simulink model "LongitudinalControl"  (R2018b)
settings: Solver=FixedStepAuto  StartTime=0.0  StopTime=100  FixedStep=0.001  RelTol=5e-3
model workspace (MAT data in the model file):
  A_mu = 10
  AxlIxx = 62.3745166667
  AxlM = 160
  B_reff = 8.386
  Cps = 2
  Cps1 = 2
  Cz = 7766.25
  Cz1 = 5565.2246438
  CzWhlAxl = 11490.971257
  DCT_Param : struct (value not decoded)
  DCT_Param1 : struct (value not decoded)
  D_reff = 0.25826
  Downshift_Speeds = [9.5625 12.9375 16.3125 19.6875 23.0625 26.4375 29.8125 33.1875 36.5625 39.9375 43.3125 46.6875 ... (28 elements, 4x7)]
  Downshift_Speeds1 = [9.5625 12.9375 16.3125 19.6875 23.0625 26.4375 29.8125 33.1875 36.5625 39.9375 43.3125 46.6875 ... (28 elements, 4x7)]
  F0z = [6086.4 4324.8]
  F0z1 = [2886 2907]
  F0zWhlAxl = 2907
  F_reff = 0.07394
  F_zmax = 10000
  F_zmin = 100
  F_zo = 4000
  Hmax = 0.25
  Kz = 48000
  Kz1 = 52451.0065793
  KzWhlAxl = 138031.612078
  MF : struct (value not decoded)
  NCyl = 6
  NCyl1 = 6
  NE_VEC = [800 1200 1600 2000 2400 2800 3200 3600 4000 4400 4800]
  Pedal_Positions = [0.1 0.4 0.5 0.9]
  Pedal_Positions1 = [0.1 0.4 0.5 0.9]
  Pstd = 101325
  Pstd1 = 101325
  Rair = 287
  Rair1 = 287
  SUS : struct (value not decoded)
  SUS1 : struct (value not decoded)
  MCOS : class17 (value not decoded)
  MCOS : class17 (value not decoded)
  MCOS : class17 (value not decoded)
  Trans : struct (value not decoded)
  Trans1 : struct (value not decoded)
  Tstd = 293.15
  Tstd1 = 293.15
  Upshift_Speeds = [12.9375 16.3125 19.6875 33 26.4375 29.8125 33.1875 52.5 39.9375 43.3125 46.6875 77.25 ... (28 elements, 4x7)]
  Upshift_Speeds1 = [12.9375 16.3125 19.6875 33 26.4375 29.8125 33.1875 52.5 39.9375 43.3125 46.6875 77.25 ... (28 elements, 4x7)]
  VEH : struct (value not decoded)
  VEH1 : struct (value not decoded)
  V_o = 16.7
  V_xlow = 1
  Vd = 0.00346
  Vd1 = 0.00346
  WH : struct (value not decoded)
  WH1 : struct (value not decoded)
  a = 1.4
  alpha_max = 1.5
  alpha_min = -1.5
  b = 1.8
  c_zo = 209651
  dt3D = 0.05
  epsilon = 0.1
  f_air = [0 0 0 0 0 0 0 0 0 0 0 0 ... (256 elements, 16x16)]
  f_air1 = [0 0 0 0 0 0 0 0 0 0 0 0 ... (256 elements, 16x16)]
  f_co = [0 0 0 0 0 0 0 0 0 0 0 0 ... (256 elements, 16x16)]
  f_co1 = [0 0 0 0 0 0 0 0 0 0 0 0 ... (256 elements, 16x16)]
  f_co2 = [0 0 0 0 0 0 0 0 0 0 0 0 ... (256 elements, 16x16)]
  f_co3 = [0 0 0 0 0 0 0 0 0 0 0 0 ... (256 elements, 16x16)]
  f_eff = [352.135682859 352.135682859 320.724378192 303.655312657 295.930136708 291.240087194 291.240271258 291.240312459 291.240275452 291.240198499 291.240100781 291.240018769 ... (256 elements, 16x16)]
  f_eff1 = [352.135682859 352.135682859 320.724378192 303.655312657 295.930136708 291.240087194 291.240271258 291.240312459 291.240275452 291.240198499 291.240100781 291.240018769 ... (256 elements, 16x16)]
  f_fuel = [0 0 0 0 0 0 0 0 0 0 0 0 ... (256 elements, 16x16)]
  f_fuel1 = [0 0 0 0 0 0 0 0 0 0 0 0 ... (256 elements, 16x16)]
  f_hc = [0 0 0 0 0 0 0 0 0 0 0 0 ... (256 elements, 16x16)]
  f_hc1 = [0 0 0 0 0 0 0 0 0 0 0 0 ... (256 elements, 16x16)]
  f_nox = [0 0 0 0 0 0 0 0 0 0 0 0 ... (256 elements, 16x16)]
  f_nox1 = [0 0 0 0 0 0 0 0 0 0 0 0 ... (256 elements, 16x16)]
  f_pm = [0 0 0 0 0 0 0 0 0 0 0 0 ... (256 elements, 16x16)]
  f_pm1 = [0 0 0 0 0 0 0 0 0 0 0 0 ... (256 elements, 16x16)]
  f_susp_axl_bp = [1 2]
  f_susp_axl_bp1 = [1 2]
  f_susp_dz_bp = [-4 -0.14 -0.13 -0.12 -0.11 -0.1 -0.09 -0.08 -0.07 -0.06 -0.05 -0.04 ... (31 elements, 1x31)]
  f_susp_dz_bp1 = [-0.325022776267 -0.315022776267 -0.305022776267 -0.205022776267 -0.105022776267 -0.00502277626717 0.0949772237328 0.194977223733 0.204977223733 0.214977223733]
  f_susp_dzdot_bp = [-4 -0.14 -0.13 -0.12 -0.11 -0.1 -0.09 -0.08 -0.07 -0.06 -0.05 -0.04 ... (31 elements, 1x31)]
  f_susp_dzdot_bp1 = [-3 -0.3 -0.2 -0.1 0 0.1 0.2 0.3 3]
  f_susp_fmz = [-213379.591456 -28099.591456 -27619.591456 -27139.591456 -26659.591456 -26179.591456 -25699.591456 -25219.591456 -24739.591456 -24259.591456 -23779.591456 -23299.591456 ... (468968 elements, 31x31x61x2x4)]
  f_susp_fmz1 = [-144070.391448 -93629.24037 -75929.1118915 -20630.5828179 -15385.48216 -10140.3815021 -4895.28084414 349.819813785 -31916.3973792 18437.6709544 -83996.1993354 -33555.0482577 ... (43920 elements, 10x9x61x2x4)]
  f_susp_geom = [-0.832564012244 0.043269987756 0.045538987756 0.047807987756 0.050076987756 0.052345987756 0.054614987756 0.056883987756 0.059152987756 0.061421987756 0.063690987756 0.065959987756 ... (11346 elements, 31x61x2x3)]
  f_susp_geom1 = [0 0 0 0 0 0 0 0 0 0 0 0 ... (3660 elements, 10x61x2x3)]
  f_susp_strgdelta_bp = [-0.523598775598 -0.506145483078 -0.488692190558 -0.471238898038 -0.453785605519 -0.436332312999 -0.418879020479 -0.401425727959 -0.383972435439 -0.366519142919 -0.349065850399 -0.331612557879 ... (61 elements, 1x61)]
  f_susp_strgdelta_bp1 = [-0.523598775598 -0.506145483078 -0.488692190558 -0.471238898038 -0.453785605519 -0.436332312999 -0.418879020479 -0.401425727959 -0.383972435439 -0.366519142919 -0.349065850399 -0.331612557879 ... (61 elements, 1x61)]
  f_tbrake = [0 76.8593923996 105.140482948 131.533638111 157.926793274 176.658631717 176.65727296 176.656856686 176.656879077 176.657093756 176.657404516 176.65772406 ... (256 elements, 16x16)]
  f_tbrake1 = [0 76.8593923996 105.140482948 131.533638111 157.926793274 176.658631717 176.65727296 176.656856686 176.656879077 176.657093756 176.657404516 176.65772406 ... (256 elements, 16x16)]
  f_tbrake_n_bpt = [0 649.519052838 912.419621844 1175.32019085 1438.22075986 1701.12132886 1964.02189787 2226.92246687 2489.82303588 2752.72360489 3015.62417389 3278.5247429 ... (16 elements, 1x16)]
  f_tbrake_n_bpt1 = [0 649.519052838 912.419621844 1175.32019085 1438.22075986 1701.12132886 1964.02189787 2226.92246687 2489.82303588 2752.72360489 3015.62417389 3278.5247429 ... (16 elements, 1x16)]
  f_tbrake_t_bpt = [0 34.6410161514 61.0341713143 87.4273264773 113.82048164 140.213636803 166.606791966 192.999947129 219.393102292 245.786257455 272.179412618 298.572567781 ... (16 elements, 1x16)]
  f_tbrake_t_bpt1 = [0 34.6410161514 61.0341713143 87.4273264773 113.82048164 140.213636803 166.606791966 192.999947129 219.393102292 245.786257455 272.179412618 298.572567781 ... (16 elements, 1x16)]
  f_texh = [766.752464599 766.752464599 786.17542386 801.679939032 884.591982581 910.574397722 910.571871054 910.570774534 910.570601632 910.570821151 910.571247242 910.571639815 ... (256 elements, 16x16)]
  f_texh1 = [766.752464599 766.752464599 786.17542386 801.679939032 884.591982581 910.574397722 910.571871054 910.570774534 910.570601632 910.570821151 910.571247242 910.571639815 ... (256 elements, 16x16)]
  f_twc_eff_co = [0.17 0.25 0.45 0.99 0.99 0.99 0.99]
  f_twc_eff_co1 = [0.17 0.25 0.45 0.99 0.99 0.99 0.99]
  f_twc_eff_hc = [0.21 0.375 0.75 0.98 0.98 0.98 0.98]
  f_twc_eff_hc1 = [0.21 0.375 0.75 0.98 0.98 0.98 0.98]
  f_twc_eff_lam = [0.909090909 0.944055944 0.979020979 1 1.013986014 1.048951049 1.083916084]
  f_twc_eff_lam1 = [0.909090909 0.944055944 0.979020979 1 1.013986014 1.048951049 1.083916084]
  f_twc_eff_nox = [0.98 0.98 0.98 0.97 0.05 0.02 0]
  f_twc_eff_nox1 = [0.98 0.98 0.98 0.97 0.05 0.02 0]
  h = 0.134
  h1 = 0.5
  h2 = 0.134
  k_z = 50
  kappa_max = 1.5
  kappa_min = -1.5
  lam_Cx = 1
  lam_Cy = 1
  lam_Cz = 1
  lam_Ex = 1
  lam_Ey = 1
  lam_F_zo = 1
  lam_Hx = 1
  lam_Hy = 1
  lam_Kxkappa = 1
  lam_Kyalpha = 1
  lam_Kygamma = 1
  lam_Kzgamma = 1
  lam_Mr = 1
  lam_Mx = 1
  lam_My = 1
  lam_S = 1
  lam_VMx = 1
  lam_Vx = 1
  lam_Vy = 1
  lam_Vykappa = 1
  lam_muV = 0
  lam_mux = 1
  lam_muy = 1
  lam_t = 1
  lam_xalpha = 1
  lam_ykappa = 1
  numWheel = 4
  numWheel1 = 4
  p_Cx1 = 1.579
  p_Cy1 = 1.3332
  p_Dx1 = 1.0422
  p_Dx2 = -0.08285
  p_Dx3 = 0
  p_Dy1 = 0.8784
  p_Dy2 = -0.06445
  p_Dy3 = 0
  p_Ex1 = 0.11185
  p_Ex2 = 0.3127
  p_Ex3 = 0
  p_Ex4 = 0.001603
  p_Ey1 = -0.8227
  p_Ey2 = -0.6062
  p_Ey3 = 0.09825
  p_Ey4 = -6.546
  p_Ey5 = 0
  p_Fz1 = 0.7098
  p_Hx1 = 0.00021585
  p_Hx2 = 0.0011538
  p_Hy1 = -0.0018043
  p_Hy2 = 0.003518
  p_Kx1 = 21.69
  p_Kx2 = 13.774
  p_Kx3 = -0.4119
  p_Ky1 = -15.314
  p_Ky2 = 1.7044
  p_Ky3 = 0.36986
  p_Ky4 = 1.9896
  p_Ky5 = 0
  p_Ky6 = -0.9004
  p_Ky7 = -0.2328
  p_Vx1 = 1.5973e-05
  p_Vx2 = 0.0001043
  p_Vy1 = -0.006642
  p_Vy2 = 0.03597
  p_Vy3 = -0.1621
  p_Vy4 = -0.4908
  p_pmx1 = 0
  p_px1 = -0.3489
  p_px2 = 0.382
  p_px3 = -0.09634
  p_px4 = 0.06447
  p_py1 = -0.6249
  p_py2 = -0.06535
  p_py3 = -0.1668
  p_py4 = 0.2834
  p_py5 = 0
  path : struct (value not decoded)
  pio = 220000
  q_Fcx = 0
  q_Fz2 = 15.4
  q_Fzy = 0
  q_reo = 0.9974
  q_sx1 = -0.007764
  q_sx10 = 0.2824
  q_sx11 = 5.349
  q_sx12 = 0
  q_sx13 = 0
  q_sx14 = 0
  q_sx2 = 1.1915
  q_sx3 = 0.013948
  q_sx4 = 4.912
  q_sx5 = 1.02
  q_sx6 = 22.83
  q_sx7 = 0.7104
  q_sx8 = -0.023393
  q_sx9 = 0.6581
  q_sy1 = 0.00702
  q_sy2 = 0
  q_sy3 = 0.001515
  q_sy4 = 8.514e-05
  q_sy5 = 0
  q_sy6 = 0
  q_sy7 = 0.9008
  q_sy8 = -0.4089
  q_v1 = 0.0007742
  q_v2 = 0.04667
  r_Bx1 = 12.531
  r_Bx2 = 9.532
  r_Bx3 = 0
  r_By1 = 10.615
  r_By2 = 7.705
  r_By3 = 3.433e-06
  r_By4 = 0
  r_Cx1 = 1.019
  r_Cy1 = 1.0585
  r_Ex1 = -0.4487
  r_Ex2 = -0.4726
  r_Ey1 = 0.3132
  r_Ey2 = 7.63e-06
  r_Hx1 = 0.0002374
  r_Hy1 = 0.011646
  r_Hy2 = 7.63e-06
  r_Vy1 = 0.05654
  r_Vy2 = 7.63e-06
  r_Vy3 = 0
  r_Vy4 = 99.9
  r_Vy5 = 2
  r_Vy6 = 15.814
  r_o = 0.3135
  vehWidth = 2
  w = 1
symbols that are objects in the model workspace (value not decoded): Trans, VEH
undefined symbols (not defined in the file): Angular, Linear, sigbuilder_block
libraries: robotlib x31, autolibutils x10, autolibshared x8, vehdynlibsuspension x7, simulink x5, vehdynlibtire x4, autolibsharedcoupling x3, vehdynlibtirecommon x3, sharedtransform x3, sim3dlib x1, vehdynlibsteering x1, autolibshareddiff x1
(part 2 of 11)

== system LongitudinalControl/Controllers ==
  note: Converts to Acceleration to Torque
      | (probably in N-m, needs to check)
  note: Determines Gear Switching
  note: Calculates Brake Pressure
      | (probably in Pascal, needs to check)
  Driver : Inport
  VehFdbk : Inport  Port=2
  Active Differential Control : Subsystem  VariantControlMode=Label  Variant=on  LabelModeActiveChoice=0
  Blank Message1 : robotlib/Blank Message  messageClass=Message  entityType=geometry_msgs/Wrench  messageType=geometry_msgs/Wrench  SampleTime=inf
      settings: SourceProductBaseCode=RO
  Blank Message2 : robotlib/Blank Message  messageClass=Message  entityType=std_msgs/Int8  messageType=std_msgs/Int8  SampleTime=inf
      settings: SourceProductBaseCode=RO
  Brake Controller : Subsystem
  Bus Assignment1 : BusAssignment  AssignedSignals=Torque.Z
  Bus Assignment2 : BusAssignment  AssignedSignals=Data
  Bus Creator{,1..2,4} (4 alike) : BusCreator  Inputs=1
  Bus Creator3 : BusCreator  Inputs=4
  Bus Selector : BusSelector  OutputSignals=Body.xdot,Wheels.kappa,Body.r
  Bus Selector1 : BusSelector  OutputSignals=Driveline.EngSpd,Driveline.PropShftSpd
  Bus Selector2 : BusSelector  OutputSignals=Accel,Brake
  Bus Selector3 : BusSelector  OutputSignals=Steer
  Engine Control Unit (ECU) : Subsystem
  Max : MinMax  Function=max  Inputs=2
  Publish1 : robotlib/Publish  topicSource=Specify your own  topic=engine_torque_cmd  messageType=geometry_msgs/Wrench  messageQueueLength=1
      settings: SourceProductBaseCode=RO
  Publish2 : robotlib/Publish  topicSource=Specify your own  topic=gear_cmd  messageType=std_msgs/Int8  messageQueueLength=1
      settings: SourceProductBaseCode=RO
  Transmission Controller : Subsystem
  Controller : Outport
  wires:
  Transmission Controller/1(Gear) -> Bus Assignment2/2, Bus Creator1/1  "GearCmd"
  Bus Selector/2 -> Brake Controller/3(kappa)  "<kappa>"
  Engine Control Unit (ECU)/1(Trq Cmd) -> Max/1
  VehFdbk/1 -> Bus Selector1/1, Bus Selector/1
  Bus Selector/1 -> Brake Controller/2(xdot)  "<xdot>"
  Bus Selector1/1 -> Transmission Controller/2(EngSpd)  "<EngSpd>"
  Bus Selector1/2 -> Transmission Controller/3(PropShaftSpd)  "<PropShftSpd>"
  Driver/1 -> Bus Selector3/1, Bus Selector2/1
  Bus Selector2/1 -> Transmission Controller/1(Acc), Engine Control Unit (ECU)/1(<Accel>)  "<Accel>"
  Bus Selector2/2 -> Brake Controller/1(BrkCmd)  "<Brake>"
  Bus Creator/1 -> Bus Creator3/1  "ECU"
  Bus Creator1/1 -> Bus Creator3/2  "Transmission"
  Bus Creator2/1 -> Bus Creator3/3  "Brake"
  Bus Creator3/1 -> Controller/1  "Controller"
  Bus Creator4/1 -> Bus Creator3/4  "Diff"
  Active Differential Control/1(DiffPrsCmd) -> Bus Creator4/1  "PrsCmd"
  Bus Selector3/1 -> Active Differential Control/2(Steer)  "<Steer>"
  Active Differential Control/2(TrqCmd) -> [DiffTrqCmd]
  Max/1 -> Bus Assignment1/2, Bus Creator/1  "EngTrqCmd"
  [DiffTrqCmd] -> Max/2
  Bus Selector/3 -> Active Differential Control/1(YawRate)  "<r>"
  Bus Assignment1/1 -> Publish1/1
  Blank Message1/1 -> Bus Assignment1/1
  Bus Assignment2/1 -> Publish2/1
  Blank Message2/1 -> Bus Assignment2/1
  Brake Controller/1(PCmd) -> Bus Creator2/1  "PCmd"

== system LongitudinalControl/Environment ==
  Blank Message : robotlib/Blank Message  messageClass=Message  entityType=geometry_msgs/Twist  messageType=geometry_msgs/Twist  SampleTime=inf
      settings: SourceProductBaseCode=RO
  Bus Assignment : BusAssignment  AssignedSignals=Linear.X,Linear.Y,Linear.Z
  Bus Creator1 : BusCreator  Inputs=2
  Constant3 : Constant  Value=0
  Constant4 : Constant  Value=0
  Constant5 : Constant  Value=0
  Friction : Constant  Value=ones(4,1).*1.0
  Ground Feedback : Subsystem  VariantControlMode=Label  Variant=on  LabelModeActiveChoice=0
  Publish : robotlib/Publish  topicSource=Specify your own  topic=wind  messageType=geometry_msgs/Twist  messageQueueLength=1
      settings: SourceProductBaseCode=RO
  Vector Concatenate : Concatenate  NumInputs=3
  Env : Outport
  wires:
  Constant5/1 -> Vector Concatenate/3, Bus Assignment/4  "Z"
  Vector Concatenate/1 -> Bus Creator1/1  "Wind"
  Constant3/1 -> Bus Assignment/2, Vector Concatenate/1  "X"
  Constant4/1 -> Bus Assignment/3, Vector Concatenate/2  "Y"
  Ground Feedback/1(Ground) -> Bus Creator1/2  "Gnd"
  Bus Creator1/1 -> Env/1
  Friction/1 -> Ground Feedback/1(Friction)
  Bus Assignment/1 -> Publish/1
  Blank Message/1 -> Bus Assignment/1

== system LongitudinalControl/Longitudinal Driver ==
  note: Longitudinal Driver has four inputs out of which
      | two are mandory:
      | Reference Longitudinal Velocity
      | Feedbacked velocity
      | Road Grade Angle (Optional)
      | Gear Ratio (Optional)
  VehRef : Inport
  VehFdbk : Inport  Port=2
  Blank Message : robotlib/Blank Message  messageClass=Message  entityType=geometry_msgs/Wrench  messageType=geometry_msgs/Wrench  SampleTime=inf
      settings: SourceProductBaseCode=RO
  Blank Message1 : robotlib/Blank Message  messageClass=Message  entityType=geometry_msgs/Wrench  messageType=geometry_msgs/Wrench  SampleTime=inf
      settings: SourceProductBaseCode=RO
  Bus Assignment : BusAssignment  AssignedSignals=Force.X
  Bus Assignment1 : BusAssignment  AssignedSignals=Force.X
  Bus Creator1 : BusCreator  Inputs=3
  Bus Selector : BusSelector  OutputSignals=Body.xdot
  Bus Selector1 : BusSelector  OutputSignals=Steer,LngRef
  Dead Zone : DeadZone  LowerValue=-0.1  UpperValue=.1  SaturateOnIntegerOverflow=on
  Ground : Ground
  Longitudinal Driver : autolibshared/Longitudinal Driver  cntrlType=Predictive  shftType=None  velUnits=m/s  gearOut=off  Kp=5  Ki=5  Kff=.1  Kg=0  VehVelVec=[0 100]  KffVec=[.1 .1]  KpVec=[10 10]  KiVec=[5 5]  KgVec=[0 0]  m=VEH.Mass  Kpt=3000  tau=.5  L=2  aR=200  bR=2.5  cR=.5  g=9.81  vnom=5  Kaw=1  tauerr=.075  tauPt=2  GearInit=0  tShift=.1  pdlVec=[0.1 0.4 0.5 0.9]  upShftTbl=[-1 12.9375 26.4375 39.9375 51.18749999999999 62.4375 72.84375 83.25;-1 16.3125 29.8125 43.3125 54.5624 65.8125 76.78125 87.75;-1 19.6875 33.1875 46.68749999999999 57.9375 69.1875 80.71875 92.25;-1 33 52.5 77.25 100.5 138.75 161.875 185]  dwnShftTbl=[1 9.5625 23.0625 36.5625 47.8125 59.0625 68.90625 78.75;1 12.9375 26.4375 39.9375 51.18749999999999 62.4375 72.84375 83.25;1 16.3125 29.8125 43.3125 54.562499 65.8125 76.78125 87.75;1 19.6875 33.1875 46.68749999999999 57.9375 69.1875 80.71875 92.25]  tClutch=.5  tRev=.5  tPark=120  aMode=2  UpGearVec="[0  1  2  3  4  5  6  7]"  DownGearVec="[1  2  3  4  5  6  7  8]"
      settings: SourceProductName=Powertrain Blockset  SourceProductBaseCode=PW
  Publish : robotlib/Publish  topicSource=Specify your own  topic=accel_in  messageType=geometry_msgs/Wrench  messageQueueLength=1
      settings: SourceProductBaseCode=RO
  Publish1 : robotlib/Publish  topicSource=Specify your own  topic=brake_in  messageType=geometry_msgs/Wrench  messageQueueLength=1
      settings: SourceProductBaseCode=RO
  Terminator3 : Terminator
  Driver : Outport
  wires:
  Ground/1 -> Longitudinal Driver/3
  Longitudinal Driver/2 -> Bus Assignment/2, Bus Creator1/2  "Accel"
  VehFdbk/1 -> Bus Selector/1
  Bus Creator1/1 -> Driver/1
  VehRef/1 -> Bus Selector1/1  "xdotref"
  Longitudinal Driver/1 -> Terminator3/1
  Bus Selector/1 -> Dead Zone/1  "<xdot>"
  Bus Selector1/2 -> Longitudinal Driver/1  "<LngRef>"
  Bus Selector1/1 -> Bus Creator1/1  "<Steer>"
  Dead Zone/1 -> Longitudinal Driver/2
  Bus Assignment/1 -> Publish/1
  Blank Message/1 -> Bus Assignment/1
  Bus Assignment1/1 -> Publish1/1
  Blank Message1/1 -> Bus Assignment1/1
  Longitudinal Driver/3 -> Bus Assignment1/2, Bus Creator1/3  "Brake"

== system LongitudinalControl/Passenger Vehicle ==
  note: pqr: V ehicle CM angular velocity about vehicle-fixed x (roll rate)-, y (pitch rate)-, z (yaw rate)- axes, respectively, in rad/s.
  Environment : Inport
  "Steer, Accelerator and Brake Inputs" : Inport  Port=2
  Controller : Inport  Port=3
  Blank Message : robotlib/Blank Message  messageClass=Message  entityType=geometry_msgs/Twist  messageType=geometry_msgs/Twist  SampleTime=inf
      settings: SourceProductBaseCode=RO
  Bus Assignment : BusAssignment  AssignedSignals=Linear.X,Linear.Y,Linear.Z,Angular.X,Angular.Y,Angular.Z
  Bus Creator2 : BusCreator  Inputs=5
  Bus Selector2 : BusSelector  OutputSignals=xdot,ydot,zdot,p,q,r
  Driveline Subsystem : Subsystem
  Engine Subsystem : Subsystem
  Publish : robotlib/Publish  topicSource=Specify your own  topic=vel  messageType=geometry_msgs/Twist  messageQueueLength=1
      settings: SourceProductBaseCode=RO
  Vehicle Body Subsystem : Subsystem
  VehFdbk : Outport
  wires:
  Bus Creator2/1 -> VehFdbk/1
  Controller/1 -> Driveline Subsystem/1(In1), Engine Subsystem/1(In1)
  Engine Subsystem/1(Engine1) -> [EngTrq], Bus Creator2/1
  [Driveline] -> Engine Subsystem/2(In2)
  Driveline Subsystem/1(Driveline1) -> Bus Creator2/2, [Driveline]
  "Steer, Accelerator and Brake Inputs"/1 -> Driveline Subsystem/2(In2)
  [EngTrq] -> Driveline Subsystem/3(In3)
  [Wheels] -> Driveline Subsystem/4(In4)
  Driveline Subsystem/2(Steering) -> Bus Creator2/3
  Vehicle Body Subsystem/2(Wheels) -> [Wheels], Bus Creator2/5
  Environment/1 -> Vehicle Body Subsystem/1(In1)
  [Driveline] -> Vehicle Body Subsystem/2(In2)
  Vehicle Body Subsystem/1(Body) -> Bus Selector2/1, Bus Creator2/4
  Blank Message/1 -> Bus Assignment/1
  Bus Assignment/1 -> Publish/1
  Bus Selector2/1 -> Bus Assignment/2  "<xdot>"
  Bus Selector2/2 -> Bus Assignment/3  "<ydot>"
  Bus Selector2/3 -> Bus Assignment/4  "<zdot>"
  Bus Selector2/4 -> Bus Assignment/5  "<p>"
  Bus Selector2/5 -> Bus Assignment/6  "<q>"
  Bus Selector2/6 -> Bus Assignment/7  "<r>"

== system LongitudinalControl/Reference Input ==
  note: Steering angle in radians
  note: Longitudinal Velocity in m/s
  Blank Message : robotlib/Blank Message  messageClass=Message  entityType=geometry_msgs/Twist  messageType=geometry_msgs/Twist  SampleTime=inf
      settings: SourceProductBaseCode=RO
  Bus Assignment : BusAssignment  AssignedSignals=Linear.X,Angular.Z
  Bus Creator : BusCreator  Inputs=2
  Bus Selector : BusSelector  Commented=on  OutputSignals=Angular.Z,Linear.X
  Publish : robotlib/Publish  topicSource=Specify your own  topic=cmd_vel  messageType=geometry_msgs/Twist  messageQueueLength=1
      settings: SourceProductBaseCode=RO
  Signal Builder : Subsystem  Tag=STV Subsys  LoadFcn=sigbuilder_block('load');  StartFcn=sigbuilder_block('start');  StopFcn=sigbuilder_block('stop');  ClipboardFcn=sigbuilder_block('clipboard');  mask(Sigbuilder block){tuvar=[0:10]}
      mask help: Simulink:masks:SigbuilderBlock_MD
      mask init:
      | if ~strcmp(get_param(bdroot(gcbh),'SimulationStatus'),'stopped') tuvar = sigbuilder_block('maskInit'); end
      settings: CopyFcn=sigbuilder_block('copy');  DeleteFcn=sigbuilder_block('delete');  ModelCloseFcn=sigbuilder_block('modelClose');  PreSaveFcn=sigbuilder_block('preSave');  PauseFcn=sigbuilder_block('pause');  ContinueFcn=sigbuilder_block('continue');  NameChangeFcn=sigbuilder_block('namechange');  OpenFcn=sigbuilder_block('open',[0 30.75 720 695.25 ]);  CloseFcn=sigbuilder_block('close');
      mask Display: plot(0, 0, 100, 100,[2, 2, 32, 32, 2], [68, 8, 8, 68, 68],[32, 2], [38, 38], [32, 19, 2],[53, 60, 44], [32, 17, 17, 2],[16, 16, 31, 31]);txt = getActiveGroup(gcbh);text(2, 100, txt,'verticalAlignment', 'top');
  Steer : Constant  Value=0.6
  Subscribe : robotlib/Subscribe  Commented=on  topicSource=Specify your own  topic=cmd_vel  messageType=geometry_msgs/Twist  sampleTime=-1  messageQueueLength=1
      settings: SourceProductBaseCode=RO
  Terminator : Terminator  Commented=on
  Ref : Outport
  wires:
  Bus Creator/1 -> Ref/1
  Subscribe/1 -> Terminator/1
  Subscribe/2 -> Bus Selector/1
  Steer/1 -> Bus Assignment/3, Bus Creator/1  "Steer"
  Signal Builder/1(Reference Velocity) -> Bus Creator/2, Bus Assignment/2  "LngRef"
  Blank Message/1 -> Bus Assignment/1
  Bus Assignment/1 -> Publish/1

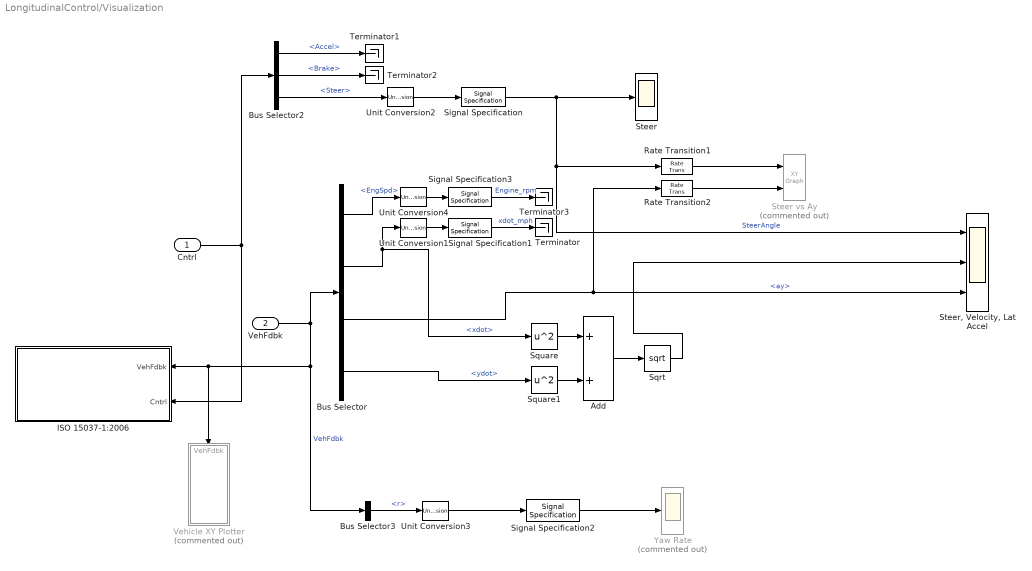
== system LongitudinalControl/Visualization ==
  Cntrl : Inport
  VehFdbk : Inport  Port=2
  Add : Sum
  Bus Selector : BusSelector  OutputSignals=Driveline.EngSpd,Body.xdot,Body.ay,Body.ydot
  Bus Selector2 : BusSelector  OutputSignals=Accel,Brake,Steer
  Bus Selector3 : BusSelector  OutputSignals=Body.r
  ISO 15037-1:2006 : Subsystem  StopFcn=|  VariantControlMode=Label  Variant=on  LabelModeActiveChoice=0  mask(ISO 15037-1:2006){Measurement=Disabled}
      | switch get_param(gcb,'Measurement')
      |     case 'Enabled'
      |        p=slproject.getCurrentProject;
      |        projectRoot=p.RootFolder;
      |        SySFolder=fullfile(projectRoot, 'System');
      |        Simulink.sdi.loadView([SySFolder filesep 'ISO15037_1_2006E.mldatx']);
      |        Simulink.sdi.view;
      | end
      mask prompts: Measurement "ISO Measurements"
      mask help: Enables display of ISO 15037-1:2006 standard measurement signals in the Simulation Data Inspector.
      mask init:
      | switch get_param(gcb,'Measurement')
      |     case 'Disabled'
      |         set_param(gcb,'OverrideUsingVariant','0')
      |     case 'Enabled'
      |        set_param(gcb,'OverrideUsingVariant','1')
      |     otherwise
      |        set_param(gcb,'OverrideUsingVariant','0')
      | end
      settings: AttributesFormatString=%<Measurement>
      mask Help: eval('vdynblkshelp(''iso15037'')');
      mask TypeOptions Measurement: Enabled | Disabled
      mask Callback Measurement:
      | switch get_param(gcb,'Measurement')
      |     case 'Disabled'
      |         set_param(gcb,'OverrideUsingVariant','0')
      |     case 'Enabled'
      |        set_param(gcb,'OverrideUsingVariant','1')
      |     otherwise
      |        set_param(gcb,'OverrideUsingVariant','0')
      | end
      mask Display: disp('ISO 15037-1:2006')
  Rate Transition1 : RateTransition  Deterministic=off  OutPortSampleTime=.1
  Rate Transition2 : RateTransition  Deterministic=off  OutPortSampleTime=.1
  Signal Specification : SignalSpecification  Unit=deg
  Signal Specification1 : SignalSpecification  Unit=mph
  Signal Specification2 : SignalSpecification  Unit=deg/s
  Signal Specification3 : SignalSpecification  Unit=rpm
  Sqrt : Sqrt  SaturateOnIntegerOverflow=on
  Square : Math  Operator=square  SaturateOnIntegerOverflow=on
  Square1 : Math  Operator=square  SaturateOnIntegerOverflow=on
  Steer : Scope
  Steer vs Ay : simulink/Sinks/XY Graph  Commented=on  xmin=-300  xmax=300  ymin=-1.5  ymax=1.5  st=.1
  "Steer, Velocity, Lat Accel" : Scope  NumInputPorts=3
  Terminator{,1..3} (4 alike) : Terminator
  Unit Conversion{1..4} (4 alike) : UnitConversion
  Vehicle XY Plotter : Subsystem  Commented=on  mask(Vehicle XY Plotter){a=VEH.FrontAxlePositionfromCG, b=VEH.RearAxlePositionfromCG, w=VEH.TrackWidth, figBorder=10, bufferSize=1024, pltDT=.1}
      mask prompts: a "Distance to front axle from CG, a [m]:"; b "Distance to rear axle from CG, b [m]:"; w "Track width, w [m]:"; figBorder "Distance to figure borders, figBorder [m]:"; bufferSize "Path buffer sampe size, bufferSize []:"; pltDT "Plot update rate, pltDT [s]:"
      mask help: This block will display a MATLAB figure which indicates the vehicle path, current position and heading velocity.
      mask TypeOptions a: Vehicle XY Plotter/a
      mask TypeOptions b: Vehicle XY Plotter/b
      mask TypeOptions w: Vehicle XY Plotter/w
      mask TypeOptions figBorder: Vehicle XY Plotter/figBorder
      mask TypeOptions bufferSize: Vehicle XY Plotter/bufferSize
  Yaw Rate : Scope  Commented=on
  wires:
  Bus Selector2/2 -> Terminator2/1  "<Brake>"
  Bus Selector/1 -> Unit Conversion4/1  "<EngSpd>"
  Cntrl/1 -> Bus Selector2/1, ISO 15037-1:2006/2(Cntrl)
  Rate Transition2/1 -> Steer vs Ay/2
  Unit Conversion2/1 -> Signal Specification/1
  Bus Selector2/1 -> Terminator1/1  "<Accel>"
  Signal Specification/1 -> Rate Transition1/1, "Steer, Velocity, Lat Accel"/1, Steer/1  "SteerAngle"
  VehFdbk/1 -> Bus Selector3/1, ISO 15037-1:2006/1(VehFdbk), Vehicle XY Plotter/1(VehFdbk), Bus Selector/1  "VehFdbk"
  Unit Conversion1/1 -> Signal Specification1/1
  Bus Selector/2 -> Square/1, Unit Conversion1/1  "<xdot>"
  Bus Selector2/3 -> Unit Conversion2/1  "<Steer>"
  Signal Specification1/1 -> Terminator/1  "xdot_mph"
  Rate Transition1/1 -> Steer vs Ay/1
  Bus Selector/3 -> Rate Transition2/1, "Steer, Velocity, Lat Accel"/3  "<ay>"
  Unit Conversion4/1 -> Signal Specification3/1
  Signal Specification3/1 -> Terminator3/1  "Engine_rpm"
  Unit Conversion3/1 -> Signal Specification2/1
  Signal Specification2/1 -> Yaw Rate/1
  Bus Selector3/1 -> Unit Conversion3/1  "<r>"
  Bus Selector/4 -> Square1/1  "<ydot>"
  Square/1 -> Add/1
  Square1/1 -> Add/2
  Add/1 -> Sqrt/1
  Sqrt/1 -> "Steer, Velocity, Lat Accel"/2

== system LongitudinalControl/Controllers/Active Differential Control ==
  note: 1) Add Subsystem or Model blocks as valid variant choices.
      | 2) You cannot connect blocks at this level. At simulation, connectivity is automatically
      | determined, based on the active variant and port name matching.
  YawRate : Inport
  Steer : Inport  Port=2
  No Control : Subsystem  VariantControl=0
  Rear Diff Controller : Subsystem  VariantControl=1
  DiffPrsCmd : Outport
  TrqCmd : Outport  Port=2

== system LongitudinalControl/Controllers/Brake Controller ==
  BrkCmd : Inport
  xdot : Inport  Port=2
  kappa : Inport  Port=3
  Abs : Abs  ZeroCross=off
  Brake Pressure Control : Subsystem  VariantControlMode=Label  Variant=on  LabelModeActiveChoice=0
  Constant1 : Constant  Value=-20
  Gain3 : Gain
  Integrator2 : Integrator  LimitOutput=on  UpperSaturationLimit=1  LowerSaturationLimit=0
  Saturation : Saturate  UpperLimit=1  LowerLimit=0  ZeroCross=off
  Switch1 : Switch  Criteria=u2 > Threshold  Threshold=.1
  Vector Concatenate2 : Concatenate  NumInputs=4
  PCmd : Outport
  wires:
  Constant1/1 -> Switch1/3
  Gain3/1 -> Switch1/1
  Saturation/1 -> Brake Pressure Control/3(<Kappa>)  "Kappa"
  Brake Pressure Control/1(PCmd) -> PCmd/1  "PCmd"
  kappa/1 -> Abs/1
  Integrator2/1 -> Vector Concatenate2/4, Vector Concatenate2/3, Vector Concatenate2/2, Vector Concatenate2/1
  xdot/1 -> Brake Pressure Control/2(xdot)
  Abs/1 -> Saturation/1
  Vector Concatenate2/1 -> Brake Pressure Control/1(Pref)  "Reference P"
  BrkCmd/1 -> Switch1/2, Gain3/1
  Switch1/1 -> Integrator2/1

== system LongitudinalControl/Controllers/Engine Control Unit (ECU) ==
  <Accel> : Inport
  Acc to Torque Request : Gain  Gain=150
  Trq Cmd : Outport
  wires:
  <Accel>/1 -> Acc to Torque Request/1
  Acc to Torque Request/1 -> Trq Cmd/1

== system LongitudinalControl/Controllers/Transmission Controller ==
  Acc : Inport
  EngSpd : Inport  Port=2  Unit=rad/s
  PropShaftSpd : Inport  Port=3
  10ms Function-Call Generator : simulink/Ports & Subsystems/Function-Call Generator  sample_time=0.05  numberOfIterations=1
  Rate Transition{,1..3} (4 alike) : RateTransition  Deterministic=off
  Signal Specification : SignalSpecification  Unit=rpm
  TCM : Subsystem
  Unit Conversion : UnitConversion
  Gear : Outport
  wires:
  TCM/1(Gear Select) -> Rate Transition3/1
  Rate Transition/1 -> TCM/1(AccCmd)
  10ms Function-Call Generator/1 -> TCM/Trigger
  Acc/1 -> Rate Transition/1
  PropShaftSpd/1 -> Rate Transition2/1
  Rate Transition1/1 -> TCM/2(EngSpd)
  Rate Transition2/1 -> TCM/3(VehSpdFdbk)
  Rate Transition3/1 -> Gear/1
  Unit Conversion/1 -> Signal Specification/1
  Signal Specification/1 -> Rate Transition1/1  "EngSpd"
  EngSpd/1 -> Unit Conversion/1

== system LongitudinalControl/Environment/Ground Feedback ==
  note: 1) Add Subsystem or Model blocks as valid variant choices.
      | 2) You cannot connect blocks at this level. At simulation, connectivity is automatically
      | determined, based on the active variant and port name matching.
  Friction : Inport
  3D Engine : Subsystem  VariantControl=1
  Constant : Subsystem  VariantControl=0
  Ground : Outport

== system LongitudinalControl/Passenger Vehicle/Driveline Subsystem ==
  In1 : Inport
  In2 : Inport  Port=2
  In3 : Inport  Port=3
  In4 : Inport  Port=4
  Driveline : Subsystem
  Subsystem1 : Subsystem
  Subsystem2 : Subsystem
  Driveline1 : Outport
  Steering : Outport  Port=2
  wires:
  Driveline/5(PropShftSpd) -> Subsystem1/5(PropShftSpd)
  Driveline/3(BrkPrs) -> Subsystem1/3(BrkPrs)
  Driveline/6(StrWhlTrq) -> Subsystem1/6(StrWhlTrq)
  Subsystem2/6(DiffPrsCmd) -> Driveline/6(DiffPrsCmd)
  Subsystem2/3(GearCmd) -> Driveline/3(GearCmd)
  Subsystem2/2(EngTrq) -> Driveline/2(EngTrq)
  Driveline/2(AxlTrq) -> Subsystem1/2(AxlTrq)
  In4/1 -> Subsystem2/4(Wheels)
  In3/1 -> Subsystem2/3(EngTrqCmd)
  In2/1 -> Subsystem2/2(SteerCmd)
  Subsystem1/2(Steering) -> Steering/1  "Steering"
  Driveline/1(WhlAng) -> Subsystem1/1(WhlAng)
  Subsystem1/1(Driveline) -> Driveline1/1  "Driveline"
  Subsystem2/1(Steer) -> Driveline/1(SteerHWCmd)
  In1/1 -> Subsystem2/1(Cntrl)
  Subsystem2/4(PrsCmd) -> Driveline/4(BrkPrsCmd)
  Subsystem2/5(omega) -> Driveline/5(omega)
  Driveline/4(EngSpd) -> Subsystem1/4(EngSpd)

== system LongitudinalControl/Passenger Vehicle/Engine Subsystem ==
  In1 : Inport
  In2 : Inport  Port=2
  Engine : Subsystem
  Subsystem3 : Subsystem
  Subsystem5 : Subsystem
  Engine1 : Outport
  wires:
  In2/1 -> Subsystem3/2(Driveline)
  In1/1 -> Subsystem3/1(Cntrl)
  Engine/1(EngTrq) -> Subsystem5/1("EngTrq ")
  Subsystem3/1(EngTrqCmd) -> Engine/1(TrqCmd)
  Subsystem3/2(EngSpd) -> Engine/2(EngSpd)
  Subsystem5/1(Eng) -> Engine1/1  "Engine"

== system LongitudinalControl/Passenger Vehicle/Vehicle Body Subsystem ==
  In1 : Inport
  In2 : Inport  Port=2
  "14DOF: Body, Suspension, Wheels" : Subsystem
  "7DOF: Body, Suspension, Wheels" : Subsystem  Commented=on
  Subsystem : Subsystem
  Subsystem4 : Subsystem
  Body : Outport
  Wheels : Outport  Port=2
  wires:
  In1/1 -> Subsystem/1(Env)
  "14DOF: Body, Suspension, Wheels"/8(GeomXYZ) -> Subsystem4/8(GeomXYZ)
  "14DOF: Body, Suspension, Wheels"/7(Beta) -> Subsystem4/7(Beta)
  "14DOF: Body, Suspension, Wheels"/1(Cgxyzdot) -> Subsystem4/1(Cgxyzdot)
  "14DOF: Body, Suspension, Wheels"/15(dzWheel) -> Subsystem4/15(dzWheel)
  In2/1 -> Subsystem/2(Driveline)
  "14DOF: Body, Suspension, Wheels"/13(XWheel) -> Subsystem4/13(XWheel)
  "14DOF: Body, Suspension, Wheels"/10(omega) -> Subsystem4/10(omega)
  Subsystem4/1(Chassis) -> Body/1  "Body"
  "14DOF: Body, Suspension, Wheels"/4(angles) -> Subsystem4/4(angles)
  Subsystem4/2(Wheels) -> Wheels/1  "Wheels"
  "14DOF: Body, Suspension, Wheels"/3(CgXYZdot) -> Subsystem4/3(CgXYZdot)
  "14DOF: Body, Suspension, Wheels"/5(pqr) -> Subsystem4/5(pqr)
  "14DOF: Body, Suspension, Wheels"/2(CgXYZ) -> Subsystem4/2(CgXYZ)
  "14DOF: Body, Suspension, Wheels"/9(GeomXYZdot) -> Subsystem4/9(GeomXYZdot)
  "14DOF: Body, Suspension, Wheels"/12(alpha) -> Subsystem4/12(alpha)
  "14DOF: Body, Suspension, Wheels"/11(kappa) -> Subsystem4/11(kappa)
  "14DOF: Body, Suspension, Wheels"/14(YWheel) -> Subsystem4/14(YWheel)
  "14DOF: Body, Suspension, Wheels"/6(Cgaxyz) -> Subsystem4/6(Cgaxyz)
  Subsystem/6(BrkPrs) -> "14DOF: Body, Suspension, Wheels"/6(BrkPrs)
  Subsystem/5(AxleTrq) -> "14DOF: Body, Suspension, Wheels"/5(AxleTrq)
  Subsystem/4(WhlAng) -> "14DOF: Body, Suspension, Wheels"/4(WheelAngle)
  Subsystem/3(mu) -> "14DOF: Body, Suspension, Wheels"/3(Friction)
  Subsystem/2(Gnd) -> "14DOF: Body, Suspension, Wheels"/2(Ground)
  Subsystem/1(Wind) -> "14DOF: Body, Suspension, Wheels"/1(WindXYZ)

== system LongitudinalControl/Reference Input/Signal Builder ==
  Demux : Demux  Tag=STV Demux  Outputs=1
  FromWs : FromWorkspace  Tag=STV FromWs  VariableName=tuvar  SampleTime=0
      SigBuilderData=|
      | common.afterFinalStr = 'Extrapolate'
      | common.sampleTime = 0
      | dataSet.timeRange = [0 100]
      | dataSet.name = 'Group 1'
      | sbobj.Groups.Name = 'Group 1'
      | sbobj.Groups.Signals.Name = 'Reference Velocity'
      | sbobj.Groups.Signals.XData = [0 6.9 12.1 15.6 20.5 24.4 28.3 31.4 36.4 40.2 44.8 50 52.7 54.9 57.9 61.6 65 72.8 75.9 78.8 82 86.4 90.5 95.1 100]
      | sbobj.Groups.Signals.YData = [0 0.338 0.632 1.354 1.67 1.945 2.515 4.18 4.61 6.85 8.7 5.84 9.68 7.88 10.94 8.42 6.6 11.8 9.1 12.14 10.25 8.55 6.6 5.65 1]
      | sbobj.Groups.TimeRange = [0 100]
  Reference Velocity : Outport  Tag=STV Outport
  wires:
  FromWs/1 -> Demux/1
  Demux/1 -> Reference Velocity/1

== system LongitudinalControl/Visualization/ISO 15037-1:2006 ==
  VehFdbk : Inport
  Cntrl : Inport  Port=2
  Disabled : Subsystem  VariantControl=0
  Enabled : Subsystem  VariantControl=1

== system LongitudinalControl/Visualization/Vehicle XY Plotter ==
  VehFdbk : Inport
  Bus Selector1 : BusSelector  OutputSignals=Body.phi,Body.theta,Body.psi  OutputAsBus=on
  Bus Selector2 : BusSelector  OutputSignals=Driveline.WhlAng  OutputAsBus=on
  Bus Selector3 : BusSelector  OutputSignals=Body.GeomX,Body.GeomY,Body.GeomZ  OutputAsBus=on
  Bus Selector4 : BusSelector  OutputSignals=Body.GeomXdot,Body.GeomYdot,Body.GeomZdot  OutputAsBus=on
  Bus to Vector{,1..3} (4 alike) : BusToVector
  Rate Transition5 : RateTransition  Deterministic=off  OutPortSampleTime=pltDT
  Vehicle XY Plotter : vehdynlibviscommon/Vehicle XY Plotter  bufferSize=bufferSize  w=w  a=a  b=b  figBorder=figBorder
  wires:
  Bus to Vector2/1 -> Vehicle XY Plotter/2  "InertCGDisp"
  Bus Selector4/1 -> Bus to Vector1/1
  Bus to Vector1/1 -> Vehicle XY Plotter/3  "InertCGVel"
  Bus Selector1/1 -> Bus to Vector2/1
  Bus to Vector/1 -> Vehicle XY Plotter/1  "InertCGDisp"
  Bus Selector3/1 -> Bus to Vector/1
  Bus Selector2/1 -> Bus to Vector3/1
  VehFdbk/1 -> Rate Transition5/1
  Bus to Vector3/1 -> Vehicle XY Plotter/4  "delta"
  Rate Transition5/1 -> Bus Selector1/1, Bus Selector2/1, Bus Selector4/1, Bus Selector3/1

== system LongitudinalControl/Controllers/Active Differential Control/No Control ==
  YawRate : Inport
  Steer : Inport  Port=2
  Ground : Ground
  Terminator : Terminator
  Terminator1 : Terminator
  Vector Concatenate2 : Concatenate  NumInputs=4
  DiffPrsCmd : Outport
  TrqCmd : Outport  Port=2
  wires:
  Ground/1 -> Vector Concatenate2/1, TrqCmd/1, Vector Concatenate2/4, Vector Concatenate2/3, Vector Concatenate2/2
  Steer/1 -> Terminator1/1
  Vector Concatenate2/1 -> DiffPrsCmd/1  "Reference P"
  YawRate/1 -> Terminator/1

== system LongitudinalControl/Controllers/Active Differential Control/Rear Diff Controller ==
  YawRate : Inport
  Steer : Inport  Port=2
  Abs : Abs  ZeroCross=off
  Abs1 : Abs  ZeroCross=off
  Cont LPF : autolibutils/Cont LPF  wc=10*pi  aMode=2
      settings: SourceProductName=Powertrain Blockset  SourceProductBaseCode=PW
  Cont LPF1 : autolibutils/Cont LPF  wc=1*pi  aMode=2
      settings: SourceProductName=Powertrain Blockset  SourceProductBaseCode=PW
  Dead Zone : DeadZone  LowerValue=-.01  UpperValue=.01  ZeroCross=off  SaturateOnIntegerOverflow=on
  Gain : Gain  Gain=1e6
  Gain2 : Gain  Gain=1/4
  Gain3 : Gain  Gain=2e3
  Ground : Ground
  Saturation : Saturate  UpperLimit=0  LowerLimit=-inf  ZeroCross=off
  Saturation1 : Saturate  UpperLimit=inf  LowerLimit=0  ZeroCross=off
  Saturation2 : Saturate  UpperLimit=1e7  LowerLimit=0  ZeroCross=off
  Saturation3 : Saturate  UpperLimit=200  LowerLimit=0  ZeroCross=off
  Subtract : Sum  Inputs=+-
  Vector Concatenate2 : Concatenate  NumInputs=4
  DiffPrsCmd : Outport
  TrqCmd : Outport  Port=2
  wires:
  Vector Concatenate2/1 -> Gain/1  "Reference P"
  Ground/1 -> Vector Concatenate2/2, Vector Concatenate2/1
  Steer/1 -> Gain2/1
  Saturation/1 -> Abs/1
  Saturation1/1 -> Vector Concatenate2/4
  Gain/1 -> Saturation2/1
  Abs/1 -> Vector Concatenate2/3
  Gain3/1 -> Saturation3/1
  Gain2/1 -> Subtract/2
  YawRate/1 -> Subtract/1
  Subtract/1 -> Dead Zone/1
  Abs1/1 -> Gain3/1
  Cont LPF/1 -> Saturation1/1, Saturation/1
  Saturation2/1 -> DiffPrsCmd/1
  Saturation3/1 -> TrqCmd/1
  Dead Zone/1 -> Cont LPF1/1, Cont LPF/1
  Cont LPF1/1 -> Abs1/1

== system LongitudinalControl/Controllers/Brake Controller/Brake Pressure Control ==
  note: 1) Add Subsystem or Model blocks as valid variant choices.
      | 2) You cannot connect blocks at this level. At simulation, connectivity is automatically
      | determined, based on the active variant and port name matching.
  Pref : Inport
  xdot : Inport  Port=2
  <Kappa> : Inport  Port=3
  Bang Bang ABS : Subsystem  VariantControl=1
  Open Loop : Subsystem  VariantControl=0
  PCmd : Outport

== system LongitudinalControl/Controllers/Transmission Controller/TCM ==
  AccCmd : Inport
  EngSpd : Inport  Port=2
  VehSpdFdbk : Inport  Port=3
  function : TriggerPort  TriggerType=function-call  VariantControl=Variant
  Neutral Select : Subsystem
  Prop Shaft Speed LPF : DiscreteTransferFcn  Numerator=[0.000000000000000 0.009950166250832 ]  Denominator=[1.000000000000000 -0.990049833749168 ]  mask(DiscretizedDiscreteTransferFcn){}
      mask init:
      | %zoh
  TCM Shift Controller : Stateflow chart  TreatAsAtomicUnit=on
  prop speed to vehicle speed : Gain  Gain=0.45
  Gear Select : Outport
  wires:
  VehSpdFdbk/1 -> Prop Shaft Speed LPF/1
  TCM Shift Controller/1(GearState) -> Gear Select/1  "GearCmd"
  AccCmd/1 -> Neutral Select/1(AccCmd), TCM Shift Controller/2(pedal)  "AccCmd"
  Neutral Select/1(Neutral Select) -> TCM Shift Controller/3(Neutral)
  EngSpd/1 -> Neutral Select/2(EngSpd)
  prop speed to vehicle speed/1 -> TCM Shift Controller/1(speed)
  Prop Shaft Speed LPF/1 -> prop speed to vehicle speed/1

== system LongitudinalControl/Environment/Ground Feedback/3D Engine ==
  Friction : Inport
  Bus Creator : BusCreator  Inputs=4
  Bus Creator2 : BusCreator  Inputs=4
  Bus Creator3 : BusCreator  Inputs=2
  Bus Selector : BusSelector  OutputSignals=HitLoc
  Data Type Conversion : DataTypeConversion
  Demux : Demux
  Demux1 : Demux
  Passenger Vehicle Ray Trace Set : sim3dlib/Vehicle Terrain Sensor  ActorTag=SimulinkVehicle1  VehExtEn=Constant  TireRadiiExt=Constant  VehCntrLngthVal=0  TireRadiiVal=0  VehRayLngth=10  LfRayLngth=20  RfRayLngth=20  LrRayLngth=20  RrRayLngth=20  VehRayOffset=0  LfRayOffset=-1  RfRayOffset=-1  LrRayOffset=-1  RrRayOffset=-1  VehEn=on  LfEn=on  RfEn=on  LrEn=on  RrEn=on  DbgEn=off  Ts=.03
  Rate Transition : RateTransition
  Reshape10 : Reshape  OutputDimensionality=Row vector (2-D)
  Selector1 : Selector  InputPortWidth=5  IndexOptions=Index vector (dialog)  Indices=[2:5]  OutputSizes=1
  Signal Specification : SignalSpecification  Unit=m
  Signal Specification1 : SignalSpecification  Unit=1
  Terminator1 : Terminator
  Terminator2 : Terminator
  Zend Select : Selector  NumberOfDimensions=2  InputPortWidth=3  IndexOptions=Select all,Index vector (dialog)  Indices=[1 3],3  OutputSizes=1,1
  Ground : Outport
  wires:
  Selector1/1 -> Rate Transition/1
  Zend Select/1 -> Reshape10/1
  Bus Selector/1 -> Zend Select/1  "<HitLoc>"
  Passenger Vehicle Ray Trace Set/2 -> Terminator1/1
  Passenger Vehicle Ray Trace Set/3 -> Terminator2/1
  Reshape10/1 -> Selector1/1
  Passenger Vehicle Ray Trace Set/1 -> Bus Selector/1
  Rate Transition/1 -> Data Type Conversion/1
  Demux/2 -> Bus Creator/2  "G_FR_z"
  Demux/1 -> Bus Creator/1  "G_FL_z"
  Demux/4 -> Bus Creator/4  "G_RR_z"
  Demux/3 -> Bus Creator/3  "G_RL_z"
  Signal Specification/1 -> Demux/1
  Signal Specification1/1 -> Demux1/1
  Demux1/1 -> Bus Creator2/1  "mu_FL"
  Bus Creator/1 -> Bus Creator3/1  "z"
  Demux1/3 -> Bus Creator2/3  "mu_RL"
  Demux1/4 -> Bus Creator2/4  "mu_RR"
  Demux1/2 -> Bus Creator2/2  "mu_FR"
  Bus Creator2/1 -> Bus Creator3/2  "mu"
  Bus Creator3/1 -> Ground/1
  Friction/1 -> Signal Specification1/1
  Data Type Conversion/1 -> Signal Specification/1

== system LongitudinalControl/Environment/Ground Feedback/Constant ==
  Friction : Inport
  Bus Creator : BusCreator  Inputs=4
  Bus Creator2 : BusCreator  Inputs=4
  Bus Creator3 : BusCreator  Inputs=2
  Constant1 : Constant  Value=zeros(4,1)
  Demux : Demux
  Demux1 : Demux
  Signal Specification : SignalSpecification  Unit=m
  Signal Specification1 : SignalSpecification  Unit=1
  Ground : Outport
  wires:
  Constant1/1 -> Signal Specification/1
  Signal Specification/1 -> Demux/1
  Demux/4 -> Bus Creator/4  "G_RR_z"
  Demux/1 -> Bus Creator/1  "G_FL_z"
  Demux/3 -> Bus Creator/3  "G_RL_z"
  Demux/2 -> Bus Creator/2  "G_FR_z"
  Bus Creator/1 -> Bus Creator3/1  "z"
  Demux1/3 -> Bus Creator2/3  "mu_RL"
  Demux1/4 -> Bus Creator2/4  "mu_RR"
  Demux1/1 -> Bus Creator2/1  "mu_FL"
  Demux1/2 -> Bus Creator2/2  "mu_FR"
  Bus Creator2/1 -> Bus Creator3/2  "mu"
  Friction/1 -> Signal Specification1/1
  Signal Specification1/1 -> Demux1/1
  Bus Creator3/1 -> Ground/1

== system LongitudinalControl/Passenger Vehicle/Driveline Subsystem/Driveline ==
  note: Copyright 2018 The MathWorks, Inc.
  SteerHWCmd : Inport
  EngTrq : Inport  Port=2
  GearCmd : Inport  Port=3  OutDataTypeStr=int8
  BrkPrsCmd : Inport  Port=4  PortDimensions=4
  omega : Inport  Port=5
  DiffPrsCmd : Inport  Port=6  PortDimensions=4
  Brake Hydraulics : Subsystem
  Ground : Ground
  Ground3 : Ground
  Kinematic Steering : vehdynlibsteering/Kinematic Steering  StrgType=Ackerman  StrgRatioType=Constant  Loc=Front  NrmlFctr=1  TrckWdth=1.922  WhlBase=(1.515+1.504)  Db=0  StrgRng=3*pi  StrgAngBpts="[-6.2832   -5.0265   -3.7699   -2.5133   -1.2566         0    1.2566    2.5133    3.7699    5.0265    6.2832]"  StrgRatioTbl=|  StrgRatio=18  StrgArmLngth=0.1  RckCsLngth=0.5  TieRodLngth=0.248128028933392  D=0.2  PnnRadius=0.0057  PnnRadiusTbl="[0.0055    0.0055    0.0056    0.0057    0.0057    0.0057    0.0057    0.0057    0.0056    0.0055    0.0055]"  RodLngth=0.1  ParaArmLngth=0.9  aMode=2
      | [13.5000   13.3750   13.2500   13.1250   13.0000   13.0000   13.0000   13.1250   13.2500   13.3750   13.5000
      | ]
      settings: SourceProductName=Vehicle Dynamics Blockset
  Prop Shaft : autolibsharedcoupling/Torsional Compliance  port_config=Simulink  k=5e3  b=100  theta_o=0  domega_o=0  omega_c=150  blkID=0  aMode=2
      settings: SourceProductName=Powertrain Blockset  SourceProductBaseCode=PW
  Subsystem : Subsystem
  Terminator : Terminator
  Terminator2 : Terminator
  Transmission : Subsystem  VariantControlMode=Label  Variant=on  LabelModeActiveChoice=0
  Vector Concatenate : Concatenate
  Vector Concatenate1 : Concatenate
  Vector Concatenate2 : Concatenate
  WhlAng : Outport  Unit=rad
  AxlTrq : Outport  Port=2
  BrkPrs : Outport  Port=3  PortDimensions=4
  EngSpd : Outport  Port=4  Unit=rad/s
  PropShftSpd : Outport  Port=5
  StrWhlTrq : Outport  Port=6  Unit=N*m
  wires:
  Kinematic Steering/3 -> Vector Concatenate/2
  Transmission/2(EngSpd) -> EngSpd/1
  GearCmd/1 -> Transmission/1(Gear)
  Ground/1 -> StrWhlTrq/1
  Transmission/1(Info) -> Terminator2/1
  Brake Hydraulics/1(BrkPrs) -> BrkPrs/1
  Kinematic Steering/2 -> Vector Concatenate/1
  Prop Shaft/2 -> Subsystem/1(DriveshfTrq)
  Kinematic Steering/1 -> Terminator/1
  SteerHWCmd/1 -> Kinematic Steering/1  "Steer"
  Subsystem/2(PropShaftSpd) -> Prop Shaft/2, PropShftSpd/1
  omega/1 -> Subsystem/2(wheels)
  Vector Concatenate2/1 -> Vector Concatenate1/2  "RearWheelAngles"
  Vector Concatenate1/1 -> WhlAng/1
  Ground3/1 -> Vector Concatenate2/2, Vector Concatenate2/1
  Vector Concatenate/1 -> Vector Concatenate1/1  "FrontWheelAngles"
  EngTrq/1 -> Transmission/2(EngTrq)
  BrkPrsCmd/1 -> Brake Hydraulics/1(BrkPrsCmd)
  Transmission/3(DiffSpd) -> Prop Shaft/1
  Prop Shaft/1 -> Transmission/3(DiffTrq)
  DiffPrsCmd/1 -> Subsystem/3(DiffPrsCmd)
  Subsystem/1(AxlTrq) -> AxlTrq/1

== system LongitudinalControl/Passenger Vehicle/Driveline Subsystem/Subsystem1 ==
  WhlAng : Inport
  AxlTrq : Inport  Port=2
  BrkPrs : Inport  Port=3
  EngSpd : Inport  Port=4
  PropShftSpd : Inport  Port=5
  StrWhlTrq : Inport  Port=6
  Bus Creator1 : BusCreator  Inputs=5
  Bus Creator2 : BusCreator  Inputs=1
  Driveline : Outport
  Steering : Outport  Port=2
  wires:
  Bus Creator1/1 -> Driveline/1  "Driveline"
  PropShftSpd/1 -> Bus Creator1/5  "PropShftSpd"
  AxlTrq/1 -> Bus Creator1/2  "AxlTrq"
  WhlAng/1 -> Bus Creator1/1  "WhlAng"
  EngSpd/1 -> Bus Creator1/4  "EngSpd"
  BrkPrs/1 -> Bus Creator1/3  "BrkPrs"
  StrWhlTrq/1 -> Bus Creator2/1  "StrWhlTrq"
  Bus Creator2/1 -> Steering/1  "Steering"

== system LongitudinalControl/Passenger Vehicle/Driveline Subsystem/Subsystem2 ==
  Cntrl : Inport
  SteerCmd : Inport  Port=2
  EngTrqCmd : Inport  Port=3
  Wheels : Inport  Port=4
  Bus Selector1 : BusSelector  OutputSignals=Steer
  Bus Selector2 : BusSelector  OutputSignals=omega
  Bus Selector3 : BusSelector  OutputSignals=Transmission.GearCmd,Brake.PCmd,Diff.PrsCmd
  Bus Selector4 : BusSelector  OutputSignals=EngTrq
  Steer : Outport
  EngTrq : Outport  Port=2
  GearCmd : Outport  Port=3
  PrsCmd : Outport  Port=4
  omega : Outport  Port=5
  DiffPrsCmd : Outport  Port=6
  wires:
  Cntrl/1 -> Bus Selector3/1
  Bus Selector3/1 -> GearCmd/1  "<GearCmd>"
  SteerCmd/1 -> Bus Selector1/1
  Wheels/1 -> Bus Selector2/1
  Bus Selector2/1 -> omega/1  "<omega>"
  EngTrqCmd/1 -> Bus Selector4/1
  Bus Selector1/1 -> Steer/1  "<Steer>"
  Bus Selector4/1 -> EngTrq/1  "<EngTrq>"
  Bus Selector3/2 -> PrsCmd/1  "<PCmd>"
  Bus Selector3/3 -> DiffPrsCmd/1  "<PrsCmd>"
